simulink model "spectrogram_model"  (R2024b)
settings: Solver=FixedStepDiscrete  StartTime=0.0  StopTime=10.0  RelTol=1e-3  EnableMultiTasking=on
undefined symbols (not defined in the file or in its folder): hw
libraries: raspberrypiAVlib x3, deeplib x1
settings Model: ExtModeTrigDuration=2  Creator=dahli  LastModifiedBy=dahli
settings SolverCC: PositivePriorityOrder=on
settings OptimizationCC: DefaultParameterBehavior=Inlined  EnhancedBackFolding=on  PassReuseOutputArgsAs=Individual arguments  ZeroExternalMemoryAtStartup=off  ZeroInternalMemoryAtStartup=off  MaxStackSize=200000  OptimizeBlockOrder=speed  DifferentSizesBufferReuse=on  OptimizationCustomize=off  EfficientTunableParamExpr=on
settings DebuggingCC: ParameterTunabilityLossMsg=error
settings HardwareCC: ProdBitPerLong=64  ProdLargestAtomicInteger=LongLong  ProdLargestAtomicFloat=Double  ProdLongLongMode=on  ProdHWDeviceType=ARM Compatible->ARM Cortex-A (64-bit)
settings RTWCC: Description=Embedded Coder  SystemTargetFile=ert.tlc  HardwareBoard=Raspberry Pi (64bit)  TLCOptions="-aInlineSetEventsForThisBaseRateFcn=TLC_FALSE -aSuppressMultiTaskScheduler=TLC_FALSE  -aRateBasedStepFcn=0"  TemplateMakefile=ert_default_tmf  Toolchain=GNU GCC Embedded Linux  BuildConfiguration=Faster Runs
settings CodeAppCC: ForceParamTrailComments=on  IgnoreCustomStorageClasses=off  OperatorAnnotations=on  SimulinkDataObjDesc=on  SFDataObjDesc=on  InsertBlockDesc=on
settings ERTTargetCC: CodeReplacementLibrary=ARM Cortex-A CMSIS  SupportVariableSizeSignals=on  ExtModeTransport=2  ExtModeStaticAlloc=on  ExtModeMexFile=ext_xcp  ExtModeIntrfLevel=Level2 - Open

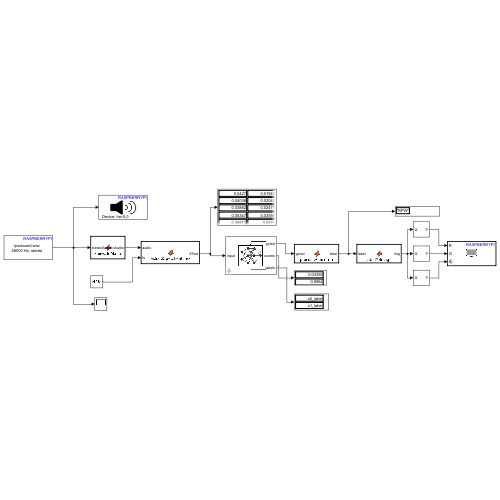
[thumbnail: Simulink's stored preview of the top-level diagram]
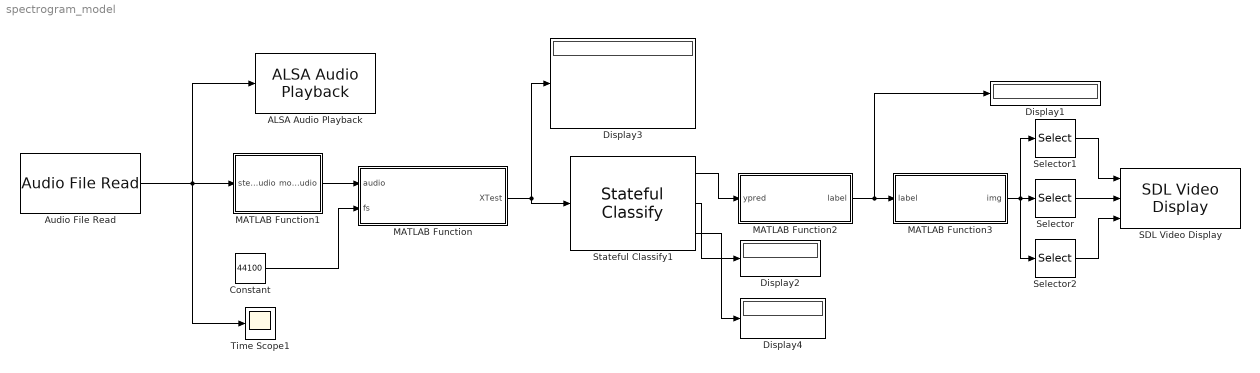
== system spectrogram_model ==
  ALSA Audio Playback : raspberrypiAVlib/ALSA Audio Playback  deviceStr=hw:0,0  sampleRateEnum=44100  queueDuration=0.5  blockPlatform=LINUX
  Audio File Read : raspberrypiAVlib/Audio File Read  FileName=C:\main\pi_recorded\rpwsound.wav  PlayCount=Inf  OutputEOFIndicator=off  SamplesPerFrame=4410
  Constant : Constant  Value=44100
  Display{1..4} (4 alike) : Display
  MATLAB Function : MATLAB Function  TreatAsAtomicUnit=on
  MATLAB Function1 : MATLAB Function  TreatAsAtomicUnit=on
  MATLAB Function2 : MATLAB Function  TreatAsAtomicUnit=on
  MATLAB Function3 : MATLAB Function  TreatAsAtomicUnit=on
  SDL Video Display : raspberrypiAVlib/SDL Video Display  title=SDL Video Display  pixelFormat=RGB  pixelOrder=Planar  rowMajor=on  blockPlatform=Raspberry Pi
  Selector : Selector  NumberOfDimensions=3  InputPortWidth=3  IndexOptions=Select all,Select all,Index vector (dialog)  Indices=[1 3],1,2  OutputSizes=1,1,1
  Selector1 : Selector  NumberOfDimensions=3  InputPortWidth=3  IndexOptions=Select all,Select all,Index vector (dialog)  Indices=[1 3],1,1  OutputSizes=1,1,1
  Selector2 : Selector  NumberOfDimensions=3  InputPortWidth=3  IndexOptions=Select all,Select all,Index vector (dialog)  Indices=[1 3],1,3  OutputSizes=1,1,1
  Stateful Classify1 : deeplib/Stateful Classify  Network=Network from MAT-file  NetworkFunction=untitled  NetworkFilePath=C:\main\rpwclassify1.mat  NetworkClassesVariable=classNames  InputDataFormats={' ',' '}  SampleTime=-1  Classification=on  Predictions=on  ForceInterpretedSim=off  PredictMode=All probabilities and labels  K=5  LastKnownNetworkFilePath=''  LastKnownNetworkTimeStamp=''
  Time Scope1 : Scope
  wires:
  Constant/1 -> MATLAB Function/2(fs)
  MATLAB Function1/1(monoAudio) -> MATLAB Function/1(audio)
  MATLAB Function/1(XTest) -> Stateful Classify1/1, Display3/1
  Audio File Read/1 -> Time Scope1/1, ALSA Audio Playback/1, MATLAB Function1/1(stereoAudio)
  Stateful Classify1/1 -> MATLAB Function2/1(ypred)
  MATLAB Function2/1(label) -> Display1/1, MATLAB Function3/1(label)
  MATLAB Function3/1(img) -> Selector2/1, Selector/1, Selector1/1
  Selector1/1 -> SDL Video Display/1
  Selector/1 -> SDL Video Display/2
  Selector2/1 -> SDL Video Display/3
  Stateful Classify1/2 -> Display2/1
  Stateful Classify1/3 -> Display4/1

== matlab function spectrogram_model/MATLAB Function1 ==
  data: stereoAudio input; monoAudio output
function monoAudio = stereoToMono(stereoAudio)
    %#codegen  
    % Ensure the input is not empty
    if isempty(stereoAudio)
        monoAudio = [];
        return;
    end
    
    % Check if the audio has two channels (stereo)
    if size(stereoAudio, 2) > 1
        % Convert to mono by averaging the two channels
        monoAudio = mean(stereoAudio, 2);
    else
        % Already mono, return as is
        monoAudio = stereoAudio;
    end
end

== matlab function spectrogram_model/MATLAB Function2 ==
  data: ypred input; label output
function label = processPrediction(ypred)
    %#codegen
    labelStr = string(ypred);

    if labelStr == "x1_label"
        label = "RPW";
    elseif labelStr == "x0_label"
        label = "NON-RPW";
    else
        label = "Unknown";
    end
end

== matlab function spectrogram_model/MATLAB Function3 ==
  data: label input; img output
function img = labelToImage(label)
%#codegen
img = uint8(zeros(240, 320, 3));
persistent rpwImage noRpwImage
if isempty(rpwImage)
    temp1 = imread('rpw_detected.jpg');
    temp2 = imread('no_rpw_detected.jpg');
    % First rotate 90 degrees to the right (clockwise)
    temp1 = rot90(temp1, -1);
    temp2 = rot90(temp2, -1);
    % Add horizontal flip to correct the text orientation
    temp1 = fliplr(temp1);
    temp2 = fliplr(temp2);
    % Then resize to [240 x 320]
    temp1 = imresize(temp1, [240 320]);
    temp2 = imresize(temp2, [240 320]);
    rpwImage = temp1;
    noRpwImage = temp2;
end
% Convert label to numeric
labelNum = 0;
if coder.target('Rtw')
    if strcmp(label, "1") || strcmp(label, "RPW")
        labelNum = 1;
    end
else
    if isequal(label, 1) || strcmp(label, "1") || strcmp(label, "RPW")
        labelNum = 1;
    end
end
% Assign correct image
if labelNum == 1
    img(:,:,:) = rpwImage;
else
    img(:,:,:) = noRpwImage;
end
end

== matlab function spectrogram_model/MATLAB Function ==
  data: audio input; XTest output; fs input
function XTest = extractSpectFeatures(audio, fs) %#codegen
    % Define Fixed Audio Length (2 sec of audio)
    fixedAudioLength = 2 * fs;  % 2 seconds of audio

    % Convert to Mono if Stereo
    if size(audio, 2) > 1
        audio = mean(audio, 2);
    end

    % Convert audio to double to avoid type mismatch
    audio = double(audio);

    % Preallocate Fixed-Length Audio (Avoid Variable-Size Issues)
    audioPadded = zeros(fixedAudioLength, 1);
    if length(audio) < fixedAudioLength
        audioPadded(1:length(audio)) = audio;
    else
        audioPadded = audio(1:fixedAudioLength);
    end
    audio = audioPadded;

    % Compute Spectrogram
    windowSize = 128; overlap = 64; nfft = 512;
    [s, ~, ~] = spectrogram(audio, windowSize, overlap, nfft, fs);

    % Convert to Magnitude Spectrogram
    spec_features = abs(s);

    % Normalize Features
    spec_features = (spec_features - min(spec_features(:))) / ...
                    (max(spec_features(:)) - min(spec_features(:)) + eps);

    % Define Fixed Feature Size (Matches Model Input)
    targetFreqBins = 257;
    targetTimeSteps = 300;
    XTest = zeros(targetFreqBins, targetTimeSteps);  % **Fixed-Size Preallocation**

    % Adjust Frequency Bins
    if size(spec_features, 1) > targetFreqBins
        spec_features = spec_features(1:targetFreqBins, :);
    elseif size(spec_features, 1) < targetFreqBins
        spec_features = [spec_features; zeros(targetFreqBins - size(spec_features, 1), size(spec_features, 2))];
    end

    % Adjust Time Steps
    if size(spec_features, 2) > targetTimeSteps
        spec_features = spec_features(:, 1:targetTimeSteps);
    elseif size(spec_features, 2) < targetTimeSteps
        spec_features = [spec_features, zeros(size(spec_features, 1), targetTimeSteps - size(spec_features, 2))];
    end

    % Assign Processed Features to Preallocated Matrix
    XTest(:,:) = spec_features;  % **Ensuring Fixed Size Output**
end
